simulink model "Phase4_Model_Student"  (R2022b)
settings: Solver=ode4  StartTime=0.0  StopTime=5  FixedStep=Ts  RelTol=1e-3
values from neighbouring files (symbols this model uses):
  A = [zeros(2,2)  eye(2) ... (first row only)    [phase4_script_Students.m]
  B = [zeros(2,1) ... (first row only)    [phase4_script_Students.m]
  C = [1 0 0 0 ... (first row only)    [phase4_script_Students.m]
  K = place(A, B, p)    [phase4_script_Students.m]
  L = transpose(L_T)    [phase4_script_Students.m]
  Ph = [0.032604651403 0.0108027150698 0.0598312321859 0.000850806189371 1.29866678626 0.0128036388307]    [ph_device_06.mat]    (also in phase4_script_Students.m = [0.0351; 0.0143; 0.0583; 0.0011; 1.7577; 0.0155])
  q10 = 0    [phase4_script_Students.m]
  q20 = pi    (= 3.14159265359)    [phase4_script_Students.m]
  X0 = [0; 0.9*pi; 0; 0]    [phase4_script_Students.m]
settings Model: Creator=shahin  LastModifiedBy=ranir
settings DataIOCC: ReturnWorkspaceOutputs=off

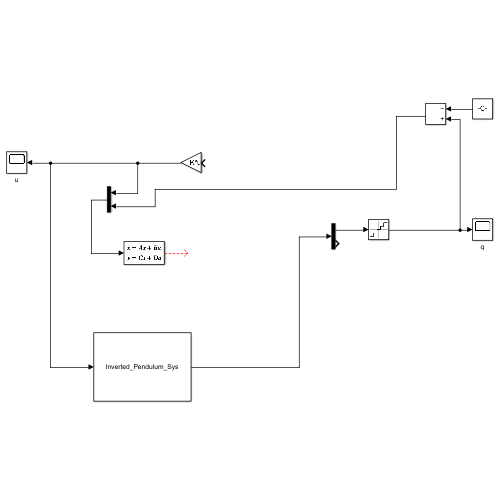
[thumbnail: Simulink's stored preview of the top-level diagram]
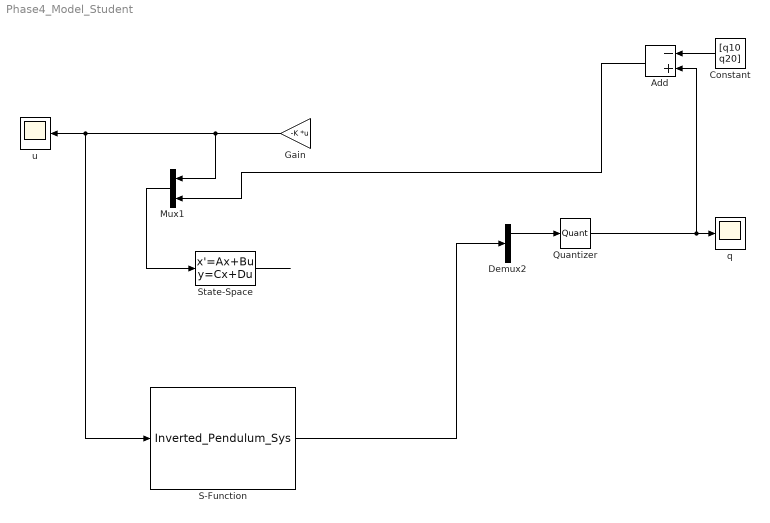
== system Phase4_Model_Student ==
  Add : Sum  Inputs=-+
  Constant : Constant  Value="[q10  q20]"
  Demux2 : Demux  Outputs=2
  Gain : Gain  Gain=-K  Multiplication=Matrix(K*u)
  Mux1 : Mux  Inputs=2
  Quantizer : Quantizer  QuantizationInterval="[2*pi/2048  2*pi/2048]"
  S-Function : S-Function  FunctionName=Inverted_Pendulum_Sys  Parameters=X0,Ph  SFunctionDeploymentMode=off  EnableBusSupport=off
  State-Space : StateSpace  A=A-L*C  B=B  C=C  D=[0;0]  InitialCondition=X0
  q : Scope
  u : Scope
  wires:
  Demux2/1 -> Quantizer/1
  S-Function/1 -> Demux2/1
  Add/1 -> Mux1/2
  Quantizer/1 -> Add/2, q/1
  Constant/1 -> Add/1
  Mux1/1 -> State-Space/1
  Gain/1 -> Mux1/1, S-Function/1, u/1
  State-Space/1 -> ?
